simulink model "pack_model"  (R2022a)
settings: Solver=VariableStepAuto  StartTime=0.0  StopTime=sim_duration  RelTol=1e-3
settings Model: Creator=Wenlin  LastModifiedBy=Wenlin

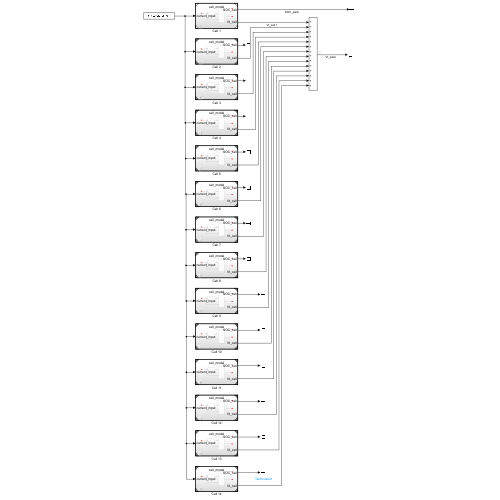
[thumbnail: Simulink's stored preview of the top-level diagram]
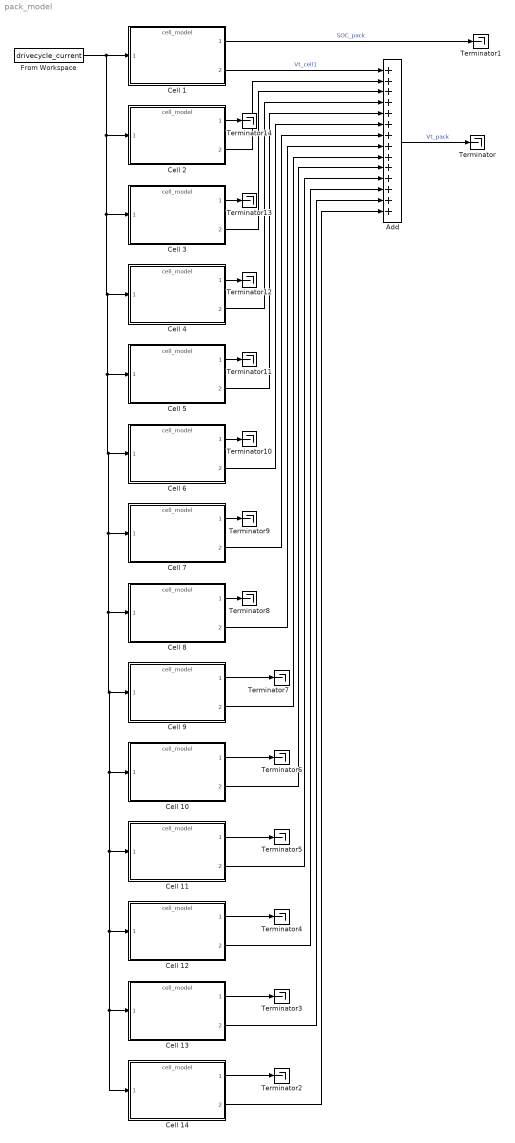
== system pack_model ==
  Add : Sum  Inputs=++++++++++++++
  Cell {1..14} (14 alike) : ModelReference  ModelNameDialog=cell_model.slx  SimulationMode=Normal  ModelReferenceVersion=1.45
  From Workspace : FromWorkspace  VariableName=drivecycle_current  OutputAfterFinalValue=Setting to zero
  Terminator{,1..14} (15 alike) : Terminator
  wires:
  From Workspace/1 -> Cell 14/1, Cell 13/1, Cell 12/1, Cell 11/1, Cell 10/1, Cell 9/1, Cell 8/1, Cell 7/1, Cell 6/1, Cell 5/1, Cell 4/1, Cell 3/1, Cell 2/1, Cell 1/1
  Cell 1/2 -> Add/1  "Vt_cell1"
  Cell 2/2 -> Add/2
  Cell 3/2 -> Add/3
  Cell 4/2 -> Add/4
  Cell 5/2 -> Add/5
  Cell 6/2 -> Add/6
  Cell 7/2 -> Add/7
  Cell 8/2 -> Add/8
  Cell 9/2 -> Add/9
  Cell 10/2 -> Add/10
  Cell 11/2 -> Add/11
  Cell 12/2 -> Add/12
  Cell 13/2 -> Add/13
  Cell 14/2 -> Add/14
  Add/1 -> Terminator/1  "Vt_pack"
  Cell 1/1 -> Terminator1/1  "SOC_pack"
  Cell 14/1 -> Terminator2/1
  Cell 13/1 -> Terminator3/1
  Cell 12/1 -> Terminator4/1
  Cell 11/1 -> Terminator5/1
  Cell 10/1 -> Terminator6/1
  Cell 9/1 -> Terminator7/1
  Cell 8/1 -> Terminator8/1
  Cell 7/1 -> Terminator9/1
  Cell 6/1 -> Terminator10/1
  Cell 5/1 -> Terminator11/1
  Cell 4/1 -> Terminator12/1
  Cell 3/1 -> Terminator13/1
  Cell 2/1 -> Terminator14/1
